simulink model "hm3_full_ascent"  (R2025b)
settings: Solver=ode45  StartTime=0  StopTime=Tstop  MaxStep=0.02  RelTol=1e-3
values from neighbouring files (symbols this model uses):
  drywind = W.drywind    [init_simulink_lpv.m]
  GreensiteLPV = L    [init_simulink_lpv.m]
  Kd_sched = Kp_sched    [init_simulink_lpv.m]
  Kp_sched = zeros(size(tsched))    [init_simulink_lpv.m]
  tsched = (o.t0:o.tsched_step:o.Tstop).'    [init_simulink_lpv.m]
undefined symbols (not defined in the file or in its folder): Kd_th0, Kd_z0, Kp_th0, Kp_z0, lpv_c1, lpv_c2, lpv_c3, lpv_c4, lpv_c5, lpv_c6, lpv_c7, lpv_invV, lpv_t, sched
libraries: simulink x2, cstblocks x1
settings Model: Creator=nickd  LastModifiedBy=nickd

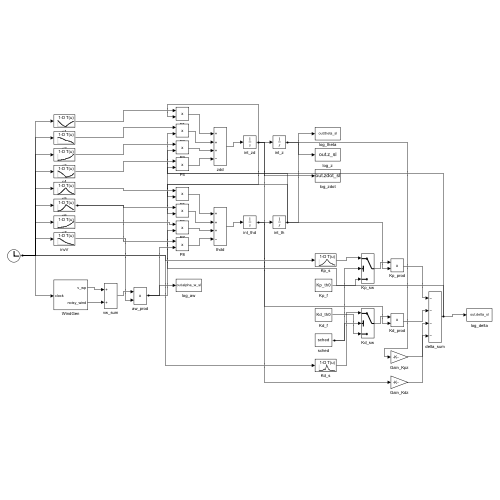
[thumbnail: Simulink's stored preview of the top-level diagram]
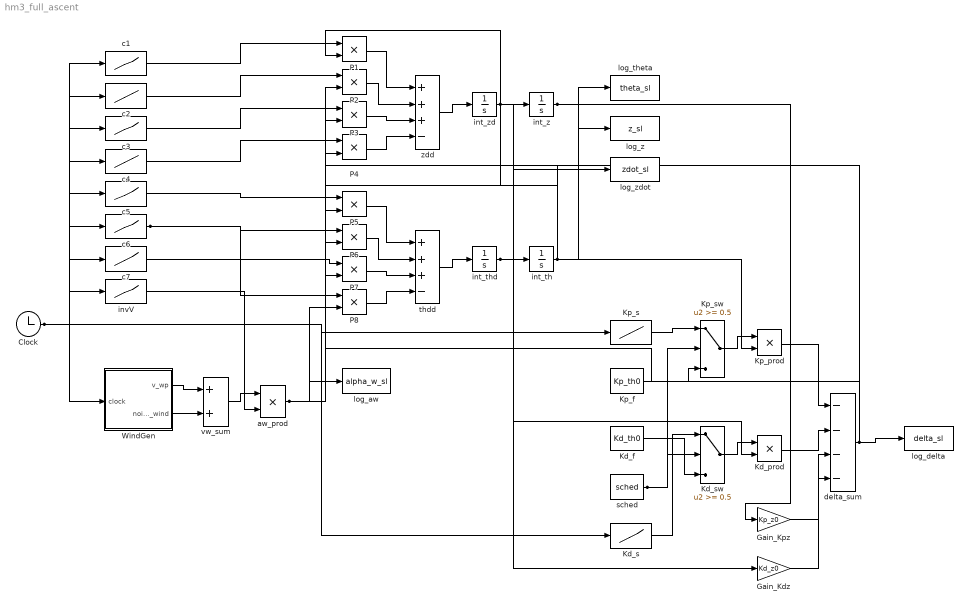
== system hm3_full_ascent ==
  Clock : Clock
  Gain_Kdz : Gain  Gain=Kd_z0
  Gain_Kpz : Gain  Gain=Kp_z0
  Kd_f : Constant  Value=Kd_th0
  Kd_prod : Product
  Kd_s : Lookup_n-D  NumberOfTableDimensions=1  BreakpointsForDimension1=tsched  BreakpointsForDimension3=[5, 7]  Table=Kd_sched  ExtrapMethod=Clip  InternalRulePriority=Speed  RndMeth=Simplest
  Kd_sw : Switch  Threshold=0.5
  Kp_f : Constant  Value=Kp_th0
  Kp_prod : Product
  Kp_s : Lookup_n-D  NumberOfTableDimensions=1  BreakpointsForDimension1=tsched  BreakpointsForDimension3=[5, 7]  Table=Kp_sched  ExtrapMethod=Clip  InternalRulePriority=Speed  RndMeth=Simplest
  Kp_sw : Switch  Threshold=0.5
  P{1..8} (8 alike) : Product
  WindGen : Subsystem
  aw_prod : Product
  c1 : Lookup_n-D  NumberOfTableDimensions=1  BreakpointsForDimension1=lpv_t  BreakpointsForDimension3=[5, 7]  Table=lpv_c1  InternalRulePriority=Speed  RndMeth=Simplest
  c2 : Lookup_n-D  NumberOfTableDimensions=1  BreakpointsForDimension1=lpv_t  BreakpointsForDimension3=[5, 7]  Table=lpv_c2  InternalRulePriority=Speed  RndMeth=Simplest
  c3 : Lookup_n-D  NumberOfTableDimensions=1  BreakpointsForDimension1=lpv_t  BreakpointsForDimension3=[5, 7]  Table=lpv_c3  InternalRulePriority=Speed  RndMeth=Simplest
  c4 : Lookup_n-D  NumberOfTableDimensions=1  BreakpointsForDimension1=lpv_t  BreakpointsForDimension3=[5, 7]  Table=lpv_c4  InternalRulePriority=Speed  RndMeth=Simplest
  c5 : Lookup_n-D  NumberOfTableDimensions=1  BreakpointsForDimension1=lpv_t  BreakpointsForDimension3=[5, 7]  Table=lpv_c5  InternalRulePriority=Speed  RndMeth=Simplest
  c6 : Lookup_n-D  NumberOfTableDimensions=1  BreakpointsForDimension1=lpv_t  BreakpointsForDimension3=[5, 7]  Table=lpv_c6  InternalRulePriority=Speed  RndMeth=Simplest
  c7 : Lookup_n-D  NumberOfTableDimensions=1  BreakpointsForDimension1=lpv_t  BreakpointsForDimension3=[5, 7]  Table=lpv_c7  InternalRulePriority=Speed  RndMeth=Simplest
  delta_sum : Sum  Inputs=----
  int_th : Integrator
  int_thd : Integrator
  int_z : Integrator
  int_zd : Integrator
  invV : Lookup_n-D  NumberOfTableDimensions=1  BreakpointsForDimension1=lpv_t  BreakpointsForDimension3=[5, 7]  Table=lpv_invV  InternalRulePriority=Speed  RndMeth=Simplest
  log_aw : ToWorkspace  VariableName=alpha_w_sl  SaveFormat=Timeseries  SampleTime=-1
  log_delta : ToWorkspace  VariableName=delta_sl  SaveFormat=Timeseries  SampleTime=-1
  log_theta : ToWorkspace  VariableName=theta_sl  SaveFormat=Timeseries  SampleTime=-1
  log_z : ToWorkspace  VariableName=z_sl  SaveFormat=Timeseries  SampleTime=-1
  log_zdot : ToWorkspace  VariableName=zdot_sl  SaveFormat=Timeseries  SampleTime=-1
  sched : Constant  Value=sched
  thdd : Sum  Inputs=+++-
  vw_sum : Sum
  zdd : Sum  Inputs=+++-
  wires:
  Clock/1 -> c1/1, c2/1, c3/1, c4/1, c5/1, c6/1, c7/1, invV/1, WindGen/1(clock), Kp_s/1, Kd_s/1
  WindGen/1(v_wp) -> vw_sum/1
  WindGen/2(noisy_wind) -> vw_sum/2
  vw_sum/1 -> aw_prod/1
  invV/1 -> aw_prod/2
  c1/1 -> P1/1
  c2/1 -> P2/1
  c3/1 -> P3/1
  c4/1 -> P4/1
  c5/1 -> P5/1
  c6/1 -> P6/1, P8/1
  c7/1 -> P7/1
  P1/1 -> zdd/1
  P2/1 -> zdd/2
  P3/1 -> zdd/3
  P4/1 -> zdd/4
  P5/1 -> thdd/1
  P6/1 -> thdd/2
  P7/1 -> thdd/3
  P8/1 -> thdd/4
  zdd/1 -> int_zd/1
  int_zd/1 -> int_z/1, P1/2, P5/2, Gain_Kdz/1, log_zdot/1
  thdd/1 -> int_thd/1
  int_thd/1 -> int_th/1, Kd_prod/2
  int_th/1 -> P2/2, P6/2, Kp_prod/2, log_theta/1
  aw_prod/1 -> P4/2, P8/2, log_aw/1
  Kp_s/1 -> Kp_sw/1
  sched/1 -> Kp_sw/2, Kd_sw/2
  Kp_f/1 -> Kp_sw/3
  Kd_s/1 -> Kd_sw/1
  Kd_f/1 -> Kd_sw/3
  Kp_sw/1 -> Kp_prod/1
  Kd_sw/1 -> Kd_prod/1
  int_z/1 -> Gain_Kpz/1, log_z/1
  Kp_prod/1 -> delta_sum/1
  Kd_prod/1 -> delta_sum/2
  Gain_Kpz/1 -> delta_sum/3
  Gain_Kdz/1 -> delta_sum/4
  delta_sum/1 -> P3/2, P7/2, log_delta/1

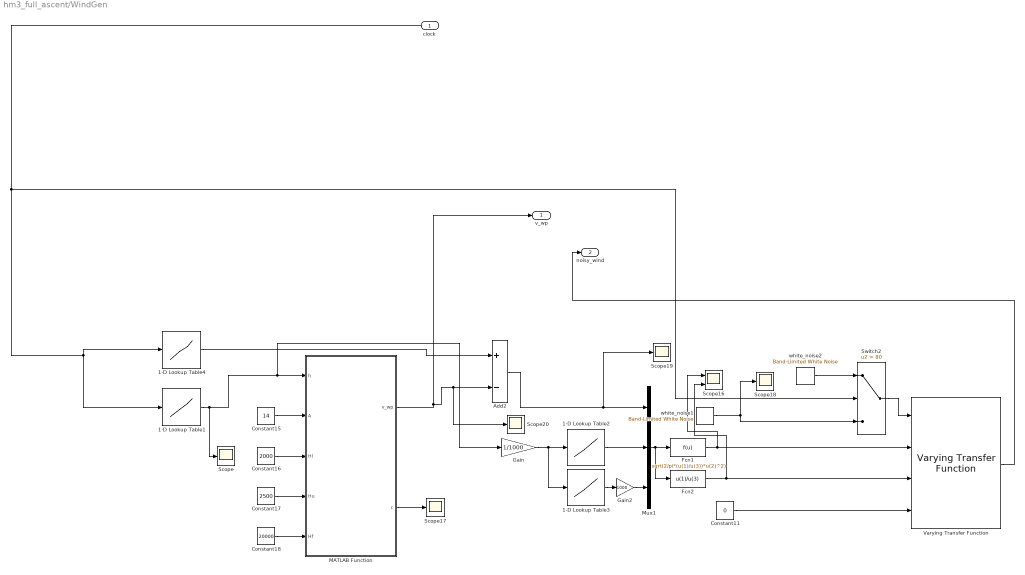
== system hm3_full_ascent/WindGen ==
  clock : Inport
  1-D Lookup Table1 : Lookup_n-D  NumberOfTableDimensions=1  BreakpointsForDimension1=GreensiteLPV.h.Time  Table=GreensiteLPV.h.Data  InternalRulePriority=Speed  RndMeth=Simplest
  1-D Lookup Table2 : Lookup_n-D  NumberOfTableDimensions=1  BreakpointsForDimension1=drywind.alt  Table=drywind.sigma.severe  InternalRulePriority=Speed  RndMeth=Simplest
  1-D Lookup Table3 : Lookup_n-D  NumberOfTableDimensions=1  BreakpointsForDimension1=drywind.alt  Table=drywind.Lh  InternalRulePriority=Speed  RndMeth=Simplest
  1-D Lookup Table4 : Lookup_n-D  NumberOfTableDimensions=1  BreakpointsForDimension1=GreensiteLPV.V.Time  Table=GreensiteLPV.V.Data  InternalRulePriority=Speed  RndMeth=Simplest
  Add2 : Sum  Inputs=+-
  Constant11 : Constant  Value=0
  Constant15 : Constant  Value=14
  Constant16 : Constant  Value=2000
  Constant17 : Constant  Value=2500
  Constant18 : Constant  Value=20000
  Fcn1 : Fcn  Expr=sqrt(2/pi*(u(1)/u(3))*u(2)^2)
  Fcn2 : Fcn  Expr=u(1)/u(3)
  Gain : Gain  Gain=1/1000
  Gain2 : Gain  Gain=1000
  MATLAB Function : MATLAB Function  TreatAsAtomicUnit=on
  Mux1 : Mux  Inputs=3
  Scope{,17..20} (5 alike) : Scope
      Scope settings: ActiveDisplayYMinimum=-1458.97416  ActiveDisplayYMaximum=2717.35091
      Scope17 settings: ActiveDisplayYMinimum=0.625  ActiveDisplayYMaximum=4.375  DataLoggingVariableName=ScopeData3
      Scope18 settings: ActiveDisplayYMinimum=-3.93527  ActiveDisplayYMaximum=3.43758  DataLoggingVariableName=ScopeData4
      Scope19 settings: ActiveDisplayYMinimum=-85.51979  ActiveDisplayYMaximum=1117.18381  DataLoggingVariableName=ScopeData5
      Scope20 settings: ActiveDisplayYMinimum=-1.75  ActiveDisplayYMaximum=15.75  DataLoggingVariableName=ScopeData6
  Scope16 : Scope  NumInputPorts=2
      settings: ActiveDisplayYMinimum=-0.02802  ActiveDisplayYMaximum=1.05151  DataLoggingVariableName=ScopeData2
  Switch2 : Switch  Criteria=u2 > Threshold  Threshold=80  SaturateOnIntegerOverflow=off  InputSameDT=off
  Varying Transfer Function : cstblocks/Linear Parameter Varying/Varying Transfer Function  N=1
      settings: SourceProductName=Control System Toolbox
  white_noise1 : simulink/Sources/Band-Limited White Noise  Cov=[1]  Ts=0.1  seed=22222
  white_noise2 : simulink/Sources/Band-Limited White Noise  Cov=[0.01]  Ts=0.1  seed=22222
  v_wp : Outport
  noisy_wind : Outport  Port=2
  wires:
  Fcn1/1 -> Scope16/1, Varying Transfer Function/2
  Constant17/1 -> MATLAB Function/4(Hu)
  Constant18/1 -> MATLAB Function/5(Hf)
  1-D Lookup Table2/1 -> Mux1/2
  Gain/1 -> 1-D Lookup Table3/1, 1-D Lookup Table2/1
  1-D Lookup Table3/1 -> Gain2/1
  Varying Transfer Function/1 -> noisy_wind/1
  Constant11/1 -> Varying Transfer Function/4
  Fcn2/1 -> Scope16/2, Varying Transfer Function/3
  Switch2/1 -> Varying Transfer Function/1
  white_noise2/1 -> Switch2/1
  MATLAB Function/2(c) -> Scope17/1
  Constant16/1 -> MATLAB Function/3(Hl)
  white_noise1/1 -> Scope18/1, Switch2/3
  Constant15/1 -> MATLAB Function/2(A)
  clock/1 -> Switch2/2, 1-D Lookup Table4/1, 1-D Lookup Table1/1
  1-D Lookup Table1/1 -> Gain/1, MATLAB Function/1(h), Scope/1
  Mux1/1 -> Fcn2/1, Fcn1/1
  Gain2/1 -> Mux1/3
  MATLAB Function/1(v_wp) -> Scope20/1, Add2/2, v_wp/1
  1-D Lookup Table4/1 -> Add2/1
  Add2/1 -> Scope19/1, Mux1/1

== matlab function hm3_full_ascent/WindGen/MATLAB Function ==
  data: h input; v_wp output; A input; Hl input; Hu input; Hf input; c output
function [v_wp,c] = fcn(h,A,Hl,Hu,Hf)
    if h < Hl
        v_wp = 10*A*(((h/2000)^(0.9))-0.9*(h/Hl));
        c = 1;
    elseif h >= Hl & h <= Hf-Hu
        v_wp = A;
        c = 2;
    elseif h > Hf-Hu & h <=Hf
        v_wp = A/2*(1 - cos((pi/Hu)*(h-Hf)));
        c = 3;
    else 
        v_wp = 0;
        c = 4;
    end
